simulink model "EgoCarModel"  (R2026a)
settings: Solver=FixedStepAuto
undefined symbols (not defined in the file): DiscIntNeverNeededParam, simulationParams, UT
libraries: sl_discontinuities x1
(part 1 of 2)
settings Model: Creator=rayyu  LastModifiedBy=rayyu

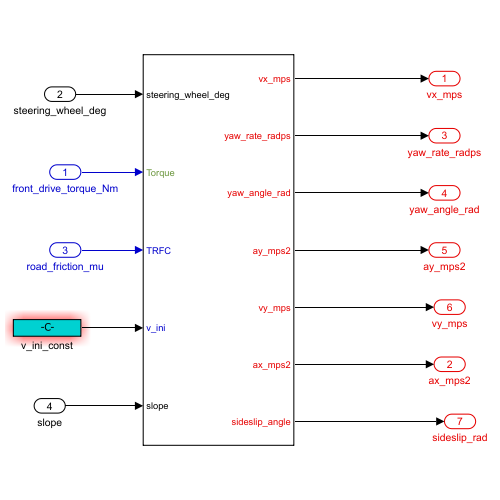
[thumbnail: Simulink's stored preview of the top-level diagram]
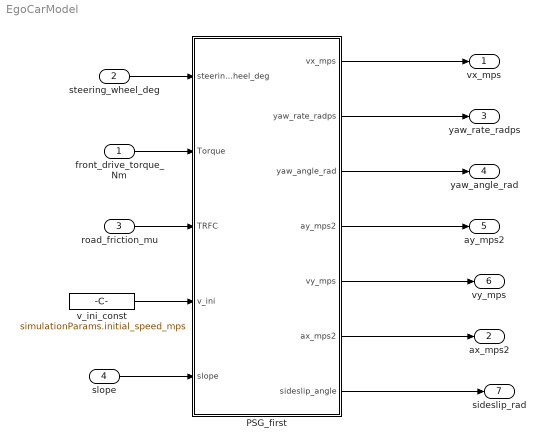
== system EgoCarModel ==
  front_drive_torque_Nm : Inport
  steering_wheel_deg : Inport  Port=2
  road_friction_mu : Inport  Port=3
  slope : Inport  Port=4
  PSG_first : Subsystem
  v_ini_const : Constant  Value=simulationParams.initial_speed_mps  VectorParams1D=off
  vx_mps : Outport
  ax_mps2 : Outport  Port=2
  yaw_rate_radps : Outport  Port=3
  yaw_angle_rad : Outport  Port=4
  ay_mps2 : Outport  Port=5
  vy_mps : Outport  Port=6
  sideslip_rad : Outport  Port=7
  wires:
  PSG_first/6(ax_mps2) -> ax_mps2/1
  road_friction_mu/1 -> PSG_first/3(TRFC)
  front_drive_torque_Nm/1 -> PSG_first/2(Torque)
  v_ini_const/1 -> PSG_first/4(v_ini)
  PSG_first/1(vx_mps) -> vx_mps/1
  steering_wheel_deg/1 -> PSG_first/1(steering_wheel_deg)
  PSG_first/2(yaw_rate_radps) -> yaw_rate_radps/1
  PSG_first/3(yaw_angle_rad) -> yaw_angle_rad/1
  PSG_first/4(ay_mps2) -> ay_mps2/1
  PSG_first/5(vy_mps) -> vy_mps/1
  PSG_first/7(sideslip_angle) -> sideslip_rad/1
  slope/1 -> PSG_first/5(slope)

== system EgoCarModel/PSG_first ==
  note: [v: 0--13--20]
      | High Frict PSG: P=75, I=125, D=15, TRFC=0.8 -->   -7.2<a<4.4
      | Low Frict  PSG: P=48, I=64,   D=12, TRFC=0.7 -->   -6.0<a<3.2
      |
      | High Frict HDV: P=27, I=27, D=9, TRFC=0.7 -->  -4.3<a<2.2
      | Low Frict  HDV: P=12, I=8,   D=6, TRFC=0.6 -->  -2.5<a<1.3
      |
      | ULMPC treat sudden drop of TRFC!
  steering_wheel_deg : Inport
  Torque : Inport  Port=2
  TRFC : Inport  Port=3
  v_ini : Inport  Port=4
  slope : Inport  Port=5
  Body Fixed Vehicle Dynamics : Subsystem
  Constant2 : Constant  Value=0
  Constant4 : Constant  Value=0
  Constant5 : Constant  Value=0
  Gain{,1..3} (4 alike) : Gain  Gain=UT.Rw
  Scope : Scope
      settings: ActiveDisplayYMinimum=-1E-6  ActiveDisplayYMaximum=1E-6
  Scope1 : Scope
      settings: ActiveDisplayYMinimum=-216705.99012  ActiveDisplayYMaximum=1.28732965782E+6  DataLoggingVariableName=ScopeData11
  Scope3 : Scope
      settings: ActiveDisplayYMinimum=-0.17988762289211868  ActiveDisplayYMaximum=0.15566007745736604  DataLoggingVariableName=ScopeData12
  Terminator : Terminator
  Vx : Scope
      settings: ActiveDisplayYMinimum=0.12308  ActiveDisplayYMaximum=39.60887  DataLoggingVariableName=ScopeData7
  ax : Scope
      settings: ActiveDisplayYMinimum=-3.96416  ActiveDisplayYMaximum=3.8969  DataLoggingVariableName=ScopeData6
  ay : Scope
      settings: ActiveDisplayYMinimum=19.63629  ActiveDisplayYMaximum=20.17019  DataLoggingVariableName=ScopeData9
  deg/rad : Gain  Gain=pi/180
  deg/rad1 : Gain  Gain=pi/180
  left/right wheel steer : Subsystem
  omegafl : Scope
      settings: ActiveDisplayYMinimum=-1.59023  ActiveDisplayYMaximum=55.33162  DataLoggingVariableName=ScopeData2
  omegafr : Scope
      settings: ActiveDisplayYMinimum=-0.02838  ActiveDisplayYMaximum=0.02291  DataLoggingVariableName=ScopeData3
  omegarl : Scope
      settings: ActiveDisplayYMinimum=-0.02838  ActiveDisplayYMaximum=0.02291  DataLoggingVariableName=ScopeData4
  omegarr : Scope
      settings: ActiveDisplayYMinimum=-0.02838  ActiveDisplayYMaximum=0.02291  DataLoggingVariableName=ScopeData5
  vy : Scope
      settings: ActiveDisplayYMinimum=19.63629  ActiveDisplayYMaximum=20.17019  DataLoggingVariableName=ScopeData10
  yaw : Scope
      settings: ActiveDisplayYMinimum=19.63629  ActiveDisplayYMaximum=20.17019
  yaw_rate : Scope
      settings: ActiveDisplayYMinimum=-0.02838  ActiveDisplayYMaximum=0.02291  DataLoggingVariableName=ScopeData8
  vx_mps : Outport
  yaw_rate_radps : Outport  Port=2
  yaw_angle_rad : Outport  Port=3
  ay_mps2 : Outport  Port=4
  vy_mps : Outport  Port=5
  ax_mps2 : Outport  Port=6
  sideslip_angle : Outport  Port=7
  wires:
  Body Fixed Vehicle Dynamics/3(omegarl) -> Gain2/1
  deg/rad1/1 -> Scope3/1, Body Fixed Vehicle Dynamics/3(deltaFR)
  Gain/1 -> omegafl/1
  Body Fixed Vehicle Dynamics/1(omegafl) -> Gain/1
  Body Fixed Vehicle Dynamics/9(ay) -> ay_mps2/1, ay/1
  v_ini/1 -> Body Fixed Vehicle Dynamics/7(V_ini)
  deg/rad/1 -> Body Fixed Vehicle Dynamics/4(deltaFL)
  slope/1 -> Body Fixed Vehicle Dynamics/5(slope)
  Body Fixed Vehicle Dynamics/12(Sideslip Angle Alpha) -> sideslip_angle/1, Scope/1
  left/right wheel steer/1(Right wheel steer ground (deg)) -> deg/rad1/1
  Body Fixed Vehicle Dynamics/10(Vy) -> vy_mps/1, vy/1
  Gain2/1 -> omegarl/1
  Body Fixed Vehicle Dynamics/8(Yaw Angle) -> yaw_angle_rad/1, yaw/1
  Body Fixed Vehicle Dynamics/11(Beta) -> Terminator/1
  Constant5/1 -> Body Fixed Vehicle Dynamics/9(vy_ini)
  steering_wheel_deg/1 -> left/right wheel steer/1(steering wheel angle deg)
  Gain3/1 -> omegarr/1
  Body Fixed Vehicle Dynamics/2(omegafr) -> Gain1/1
  Constant4/1 -> Body Fixed Vehicle Dynamics/2(Brake)
  Body Fixed Vehicle Dynamics/4(omegarr) -> Gain3/1
  Body Fixed Vehicle Dynamics/6(Vx) -> vx_mps/1, Vx/1
  Body Fixed Vehicle Dynamics/5(ax) -> ax_mps2/1, ax/1
  Constant2/1 -> Body Fixed Vehicle Dynamics/8(yaw_ini)
  left/right wheel steer/2(Left wheel steer ground (deg)) -> deg/rad/1
  Gain1/1 -> omegafr/1
  Body Fixed Vehicle Dynamics/7("Yaw Rate ") -> yaw_rate_radps/1, yaw_rate/1
  Torque/1 -> Body Fixed Vehicle Dynamics/1(Tdf), Scope1/1
  TRFC/1 -> Body Fixed Vehicle Dynamics/6(TRFC)

== system EgoCarModel/PSG_first/Body Fixed Vehicle Dynamics ==
  Tdf : Inport
  Brake : Inport  Port=2
  deltaFR : Inport  Port=3
  deltaFL : Inport  Port=4
  slope : Inport  Port=5
  TRFC : Inport  Port=6
  V_ini : Inport  Port=7
  yaw_ini : Inport  Port=8
  vy_ini : Inport  Port=9
  8dof_vehicle : Subsystem
  Brakes : Subsystem
  Bus Creator{,2..4} (4 alike) : BusCreator  Inputs=4
  Bus Creator1 : BusCreator  Inputs=8
  Bus Creator5 : BusCreator  Inputs=3
  Bus Selector : BusSelector  OutputSignals=signal1,signal2,signal3,signal4
  Constant : Constant  Value=0
  Constant1 : Constant  Value=0
  Driving Resistance Subsystem : Subsystem
  Fz : Subsystem
  Magic Formula Tire Model1 : Subsystem
  "Tire Longitudinal Center Speed " : Subsystem
  Tire Sideslip Angle : Subsystem
  To Workspace : ToWorkspace  VariableName=PSG1_FxFL  SaveFormat=Timeseries  SampleTime=-1
  To Workspace1 : ToWorkspace  VariableName=PSG1_FxRL  SaveFormat=Timeseries  SampleTime=-1
  To Workspace2 : ToWorkspace  VariableName=PSG1_FxFR  SaveFormat=Timeseries  SampleTime=-1
  To Workspace3 : ToWorkspace  VariableName=PSG1_FxRR  SaveFormat=Timeseries  SampleTime=-1
  Unit Delay : UnitDelay  SampleTime=UT.Ts_Veh
  Unit Delay1 : UnitDelay  SampleTime=UT.Ts_Veh
  deltaFL1 : InportShadow  Port=4
  deltaFL2 : InportShadow  Port=4
  deltaFR1 : InportShadow  Port=3
  deltaFR2 : InportShadow  Port=3
  lamda slip ratio : Subsystem
  omegafl : Outport  VectorParamsAs1DForOutWhenUnconnected=off
  omegafr : Outport  Port=2  VectorParamsAs1DForOutWhenUnconnected=off
  omegarl : Outport  Port=3  VectorParamsAs1DForOutWhenUnconnected=off
  omegarr : Outport  Port=4  VectorParamsAs1DForOutWhenUnconnected=off
  ax : Outport  Port=5  VectorParamsAs1DForOutWhenUnconnected=off
  Vx : Outport  Port=6  VectorParamsAs1DForOutWhenUnconnected=off
  "Yaw Rate " : Outport  Port=7  VectorParamsAs1DForOutWhenUnconnected=off
  Yaw Angle : Outport  Port=8  VectorParamsAs1DForOutWhenUnconnected=off
  ay : Outport  Port=9  VectorParamsAs1DForOutWhenUnconnected=off
  Vy : Outport  Port=10  VectorParamsAs1DForOutWhenUnconnected=off
  Beta : Outport  Port=11  VectorParamsAs1DForOutWhenUnconnected=off
  Sideslip Angle Alpha : Outport  Port=12  VectorParamsAs1DForOutWhenUnconnected=off
  wires:
  Brakes/4(Tbrr) -> 8dof_vehicle/5(Tbrr)
  Brakes/3(Tbrl) -> 8dof_vehicle/4(Tbrl)
  Brakes/2(Tbfr) -> 8dof_vehicle/3(Tbfr)
  Brakes/1(Tbfl) -> 8dof_vehicle/2(Tbfl)
  Brake/1 -> Brakes/2(brake postion)
  8dof_vehicle/14("Roll ") -> Fz/7(roll angle)
  8dof_vehicle/12(Pitch) -> Fz/4(pitch angle)
  8dof_vehicle/13(Pitch_rate) -> Fz/8(pitch rate)
  Bus Creator3/1 -> Bus Creator5/2
  deltaFR2/1 -> 8dof_vehicle/11(deltaRL)
  deltaFR1/1 -> Tire Sideslip Angle/5(deltaFR1)
  deltaFR/1 -> lamda slip ratio/10(deltaFR)
  lamda slip ratio/4(lamdarr) -> Bus Creator2/4
  lamda slip ratio/3(lamdarl) -> Bus Creator2/3
  lamda slip ratio/2(lamdafr) -> Bus Creator2/2
  lamda slip ratio/1(lamdafl) -> Bus Creator2/1
  Unit Delay/1 -> Fz/2(ax)
  Unit Delay1/1 -> Fz/5(ay)
  Magic Formula Tire Model1/4(Fy_FR) -> Bus Creator1/4
  Magic Formula Tire Model1/3(Fx_FR) -> Bus Creator1/3, To Workspace2/1
  Magic Formula Tire Model1/6(Fy_RL) -> Bus Creator1/6
  Magic Formula Tire Model1/8(Fy_RR) -> Bus Creator1/8
  Magic Formula Tire Model1/7(Fx_RR) -> Bus Creator1/7, To Workspace3/1
  Magic Formula Tire Model1/5(Fx_RL) -> Bus Creator1/5, To Workspace1/1
  deltaFL2/1 -> 8dof_vehicle/10(deltaFL)  "deltaw"
  8dof_vehicle/5(ax) -> Unit Delay/1, ax/1
  Constant/1 -> Fz/3(slope)
  Driving Resistance Subsystem/1(Fax) -> 8dof_vehicle/7(Fax), Fz/1(Fa)  "Fax"
  Constant1/1 -> Fz/6(bank angle)
  slope/1 -> 8dof_vehicle/9(slope)
  8dof_vehicle/7(Yaw Rate) -> "Tire Longitudinal Center Speed "/3(YawRate), Tire Sideslip Angle/2(Yaw Rate), "Yaw Rate "/1
  8dof_vehicle/6(Vx) -> "Tire Longitudinal Center Speed "/1(Vx), Tire Sideslip Angle/3(Vx), Driving Resistance Subsystem/1(Vx), Vx/1
  8dof_vehicle/11("Veh Sideslip, Beta") -> Tire Sideslip Angle/6(Beta), Beta/1, "Tire Longitudinal Center Speed "/4(VehSideSlip Beta)
  8dof_vehicle/9(ay) -> Unit Delay1/1, ay/1
  deltaFL1/1 -> Tire Sideslip Angle/4(deltaFL)  "deltaw"
  deltaFL/1 -> lamda slip ratio/9(deltaFL)  "deltaw"
  Driving Resistance Subsystem/2(Fr) -> 8dof_vehicle/8(Fr)
  Bus Selector/4 -> lamda slip ratio/8(Vwrr)  "<signal4>"
  Bus Selector/3 -> lamda slip ratio/7(Vwrl)  "<signal3>"
  Bus Selector/2 -> lamda slip ratio/6(Vwfr)  "<signal2>"
  Bus Selector/1 -> lamda slip ratio/5(Vwfl)  "<signal1>"
  "Tire Longitudinal Center Speed "/3(Vwrl) -> Bus Creator/3
  "Tire Longitudinal Center Speed "/1(Vwfl) -> Bus Creator/1
  "Tire Longitudinal Center Speed "/2(Vwfr) -> Bus Creator/2
  "Tire Longitudinal Center Speed "/4(Vwrr) -> Bus Creator/4
  Tire Sideslip Angle/2(alpha_fr: rad) -> Bus Creator4/2
  Tire Sideslip Angle/1(alpha_fl: rad) -> Sideslip Angle Alpha/1, Bus Creator4/1
  Tire Sideslip Angle/3(alpha_rl: rad) -> Bus Creator4/3
  Tire Sideslip Angle/4(alpha_rr: rad) -> Bus Creator4/4
  Bus Creator5/1 -> Magic Formula Tire Model1/1(VehState)
  Bus Creator4/1 -> Bus Creator5/3  "alpha"
  Bus Creator2/1 -> Brakes/1(lambda), Bus Creator5/1  "lamda"
  Fz/1(Fzfl) -> Bus Creator3/1
  Fz/2(Fzfr) -> Bus Creator3/2
  Fz/3(Fzrl) -> Bus Creator3/3
  Fz/4(Fzrr) -> Bus Creator3/4
  Magic Formula Tire Model1/1(Fx_FL) -> Bus Creator1/1, To Workspace/1
  Magic Formula Tire Model1/2(Fy_FL) -> Bus Creator1/2
  8dof_vehicle/10(Vy) -> "Tire Longitudinal Center Speed "/2(Vy), Tire Sideslip Angle/1(Vy), Vy/1
  Bus Creator1/1 -> 8dof_vehicle/6(In7)
  8dof_vehicle/8(Yaw angle) -> Yaw Angle/1
  8dof_vehicle/4(omegarr) -> lamda slip ratio/4(omegarr), omegarr/1
  8dof_vehicle/3(omegarl) -> lamda slip ratio/3(omegarl), omegarl/1
  8dof_vehicle/2(omegafr) -> omegafr/1, lamda slip ratio/2(omegafr)
  8dof_vehicle/1(omegafl) -> lamda slip ratio/1(omegafl), omegafl/1
  Tdf/1 -> 8dof_vehicle/1(Tdf)
  Bus Creator/1 -> Bus Selector/1
  TRFC/1 -> Magic Formula Tire Model1/2(TRFC)
  V_ini/1 -> 8dof_vehicle/12(V_ini)
  yaw_ini/1 -> 8dof_vehicle/13(yaw_ini)
  vy_ini/1 -> 8dof_vehicle/14(vy_ini)
  8dof_vehicle/15(Roll Rate) -> Fz/9(roll rate)

== system EgoCarModel/PSG_first/left//right wheel steer ==
  steering wheel angle deg : Inport
  Deadband Deg : DeadZone  LowerValue=-2  UpperValue=2
  Gain : Gain  Gain=0.9
  Gain1 : Gain  Gain=0.9
  Left wheel rack displacement to ground steering angle1 : Lookup_n-D  NumberOfTableDimensions=1  BreakpointsForDimension1=|  Table=|  RndMeth=Simplest
      | [-83.31
      | -80.10576923
      | -77.13888889
      | -74.38392857
      | -71.81896552
      | -69.425
      | -67.18548387
      | -65.0859375
      | -63.11363636
      | -61.25735294
      | -59.50714286
      | -57.85416667
      | -56.29054054
      | -54.80921053
      | -53.40384615
      | -52.06875
      | -50.79878049
      | -49.58928571
      | -48.43604651
      | -47.33522727
      | -46.28333333
      | -45.27717391
      | -44.31382979
      | -43.390625
      | -42.50510204
      | -41.655
      | 0
      | 41.655
      | 42.50510204
      | 43.390625
      | 44.31382979
      | 45.27717391
      | 46.28333333
      | 47.33522727
      | 48.43604651
      | 49.58928571
      | 50.79878049
      | 52.06875
      | 53.40384615
      | 54.80921053
      | 56.29054054
      | 57.85416667
      | 59.50714286
      | 61.25735294
      | 63.11363636
      | 65.0859375
      | 67.18548387
      | 69.425
      | 71.81896552
      | 74.38392857
      | 77.13888889
      | 80.10576923
      | 83.31
      | ]
      | [-39.37720355
      | -37.63494871
      | -36.07707064
      | -34.67025898
      | -33.38971041
      | -32.21639355
      | -31.13534711
      | -30.13457154
      | -29.20427963
      | -28.33637359
      | -27.52407048
      | -26.76162747
      | -26.04413644
      | -25.36736764
      | -24.72764882
      | -24.12177053
      | -23.54691095
      | -23.00057556
      | -22.48054833
      | -21.98485165
      | -21.51171342
      | -21.05953958
      | -20.62689117
      | -20.21246499
      | -19.81507719
      | -19.43364926
      | 0
      | 23.71741561
      | 24.27669186
      | 24.86323253
      | 25.47909206
      | 26.1265372
      | 26.80807528
      | 27.52648702
      | 28.28486498
      | 29.08665866
      | 29.93572777
      | 30.83640531
      | 31.7935729
      | 32.81275112
      | 33.9002085
      | 35.06309421
      | 36.30960068
      | 37.64916478
      | 39.09271935
      | 40.65301137
      | 42.34501024
      | 44.1864403
      | 46.19848973
      | 48.40677775
      | 50.84271532
      | 53.54549481
      | 56.56514507
      | ]
  Right wheel rack displacement to ground steering angle : Lookup_n-D  NumberOfTableDimensions=1  BreakpointsForDimension1=|  Table=|  RndMeth=Simplest
      | [-83.31
      | -80.10576923
      | -77.13888889
      | -74.38392857
      | -71.81896552
      | -69.425
      | -67.18548387
      | -65.0859375
      | -63.11363636
      | -61.25735294
      | -59.50714286
      | -57.85416667
      | -56.29054054
      | -54.80921053
      | -53.40384615
      | -52.06875
      | -50.79878049
      | -49.58928571
      | -48.43604651
      | -47.33522727
      | -46.28333333
      | -45.27717391
      | -44.31382979
      | -43.390625
      | -42.50510204
      | -41.655
      | 0
      | 41.655
      | 42.50510204
      | 43.390625
      | 44.31382979
      | 45.27717391
      | 46.28333333
      | 47.33522727
      | 48.43604651
      | 49.58928571
      | 50.79878049
      | 52.06875
      | 53.40384615
      | 54.80921053
      | 56.29054054
      | 57.85416667
      | 59.50714286
      | 61.25735294
      | 63.11363636
      | 65.0859375
      | 67.18548387
      | 69.425
      | 71.81896552
      | 74.38392857
      | 77.13888889
      | 80.10576923
      | 83.31
      | ]
      | [-56.56514507
      | -53.54549481
      | -50.84271532
      | -48.40677775
      | -46.19848973
      | -44.1864403
      | -42.34501024
      | -40.65301137
      | -39.09271935
      | -37.64916478
      | -36.30960068
      | -35.06309421
      | -33.9002085
      | -32.81275112
      | -31.7935729
      | -30.83640531
      | -29.93572777
      | -29.08665866
      | -28.28486498
      | -27.52648702
      | -26.80807528
      | -26.1265372
      | -25.47909206
      | -24.86323253
      | -24.27669186
      | -23.71741561
      | 0
      | 19.43364926
      | 19.81507719
      | 20.21246499
      | 20.62689117
      | 21.05953958
      | 21.51171342
      | 21.98485165
      | 22.48054833
      | 23.00057556
      | 23.54691095
      | 24.12177053
      | 24.72764882
      | 25.36736764
      | 26.04413644
      | 26.76162747
      | 27.52407048
      | 28.33637359
      | 29.20427963
      | 30.13457154
      | 31.13534711
      | 32.21639355
      | 33.38971041
      | 34.67025898
      | 36.07707064
      | 37.63494871
      | 39.37720355
      | ]
  steering wheel angle (pinion) to rack dispacement : Lookup_n-D  NumberOfTableDimensions=1  BreakpointsForDimension1=|  Table=|  RndMeth=Simplest
      BreakpointsForDimension1=|
      | [-807.1596203
      | -767.526082
      | -732.1745847
      | -700.3549602
      | -671.5005069
      | -645.1711331
      | -621.017417
      | -598.7568399
      | -578.1574816
      | -559.0264878
      | -541.2017003
      | -524.5454483
      | -508.9398532
      | -494.2832202
      | -480.4872231
      | -467.4746805
      | -455.1777777
      | -443.5366317
      | -432.4981203
      | -422.0149202
      | -412.0447096
      | -402.5495034
      | -393.495094
      | -384.8505798
      | -376.5879637
      | -368.6818104
      | 0
      | 368.6818104
      | 376.5879637
      | 384.8505798
      | 393.495094
      | 402.5495034
      | 412.0447096
      | 422.0149202
      | 432.4981203
      | 443.5366317
      | 455.1777777
      | 467.4746805
      | 480.4872231
      | 494.2832202
      | 508.9398532
      | 524.5454483
      | 541.2017003
      | 559.0264878
      | 578.1574816
      | 598.7568399
      | 621.017417
      | 645.1711331
      | 671.5005069
      | 700.3549602
      | 732.1745847
      | 767.526082
      | 807.1596203
      | ]
      Table=|
      | [-83.31
      | -80.10576923
      | -77.13888889
      | -74.38392857
      | -71.81896552
      | -69.425
      | -67.18548387
      | -65.0859375
      | -63.11363636
      | -61.25735294
      | -59.50714286
      | -57.85416667
      | -56.29054054
      | -54.80921053
      | -53.40384615
      | -52.06875
      | -50.79878049
      | -49.58928571
      | -48.43604651
      | -47.33522727
      | -46.28333333
      | -45.27717391
      | -44.31382979
      | -43.390625
      | -42.50510204
      | -41.655
      | 0
      | 41.655
      | 42.50510204
      | 43.390625
      | 44.31382979
      | 45.27717391
      | 46.28333333
      | 47.33522727
      | 48.43604651
      | 49.58928571
      | 50.79878049
      | 52.06875
      | 53.40384615
      | 54.80921053
      | 56.29054054
      | 57.85416667
      | 59.50714286
      | 61.25735294
      | 63.11363636
      | 65.0859375
      | 67.18548387
      | 69.425
      | 71.81896552
      | 74.38392857
      | 77.13888889
      | 80.10576923
      | 83.31
      | ]
  Right wheel steer ground (deg) : Outport  VectorParamsAs1DForOutWhenUnconnected=off
  Left wheel steer ground (deg) : Outport  Port=2  VectorParamsAs1DForOutWhenUnconnected=off
  wires:
  Deadband Deg/1 -> steering wheel angle (pinion) to rack dispacement/1
  Gain1/1 -> Left wheel steer ground (deg)/1
  Gain/1 -> Right wheel steer ground (deg)/1
  Left wheel rack displacement to ground steering angle1/1 -> Gain1/1
  Right wheel rack displacement to ground steering angle/1 -> Gain/1
  steering wheel angle (pinion) to rack dispacement/1 -> Right wheel rack displacement to ground steering angle/1, Left wheel rack displacement to ground steering angle1/1
  steering wheel angle deg/1 -> Deadband Deg/1

== system EgoCarModel/PSG_first/Body Fixed Vehicle Dynamics/8dof_vehicle ==
  Tdf : Inport
  Tbfl : Inport  Port=2
  Tbfr : Inport  Port=3
  Tbrl : Inport  Port=4
  Tbrr : Inport  Port=5
  In7 : Inport  Port=6
  Fax : Inport  Port=7
  Fr : Inport  Port=8
  slope : Inport  Port=9
  deltaFL : Inport  Port=10
  deltaRL : Inport  Port=11
  V_ini : Inport  Port=12
  yaw_ini : Inport  Port=13
  vy_ini : Inport  Port=14
  4tyre_torque : Subsystem
  Bus Selector1 : BusSelector  OutputSignals=Fx_FL,Fx_FR,Fx_RL,Fx_RR,Fy_FL,Fy_FR
  Bus Selector2 : BusSelector  OutputSignals=Fy_FL,Fy_FR,Fy_RL,Fy_RR,Fx_FL,Fx_FR
  Bus Selector3 : BusSelector  OutputSignals=Fx_FL,Fx_FR,Fx_RL,Fx_RR
  Bus Selector4 : BusSelector  OutputSignals=Fy_FL,Fy_FR,Fy_RL,Fy_RR,Fx_FL,Fx_FR,Fx_RL,Fx_RR
  Constant1 : Constant  Value=0
  Gain2 : Gain  Gain=-1
  "Pitch " : Subsystem
  Roll : Subsystem
  Switch{,1..3} (4 alike) : Switch  SaturateOnIntegerOverflow=off  InputSameDT=off
  Yaw Dynamics : Subsystem
  deltaFL1 : InportShadow  Port=10
  deltaFL2 : InportShadow  Port=10
  deltaRL1 : InportShadow  Port=11
  deltaRL2 : InportShadow  Port=11
  lateral : Subsystem
  longitudinal : Subsystem
  omegafl : Outport  VectorParamsAs1DForOutWhenUnconnected=off
  omegafr : Outport  Port=2  VectorParamsAs1DForOutWhenUnconnected=off
  omegarl : Outport  Port=3  VectorParamsAs1DForOutWhenUnconnected=off
  omegarr : Outport  Port=4  VectorParamsAs1DForOutWhenUnconnected=off
  ax : Outport  Port=5  VectorParamsAs1DForOutWhenUnconnected=off
  Vx : Outport  Port=6  VectorParamsAs1DForOutWhenUnconnected=off
  Yaw Rate : Outport  Port=7  VectorParamsAs1DForOutWhenUnconnected=off
  Yaw angle : Outport  Port=8  VectorParamsAs1DForOutWhenUnconnected=off
  ay : Outport  Port=9  VectorParamsAs1DForOutWhenUnconnected=off
  Vy : Outport  Port=10  VectorParamsAs1DForOutWhenUnconnected=off
  "Veh Sideslip, Beta" : Outport  Port=11  VectorParamsAs1DForOutWhenUnconnected=off
  Pitch : Outport  Port=12  VectorParamsAs1DForOutWhenUnconnected=off
  Pitch_rate : Outport  Port=13  VectorParamsAs1DForOutWhenUnconnected=off
  "Roll " : Outport  Port=14  VectorParamsAs1DForOutWhenUnconnected=off
  Roll Rate : Outport  Port=15  VectorParamsAs1DForOutWhenUnconnected=off
  wires:
  Switch/1 -> 4tyre_torque/4(Tbrl)
  Switch1/1 -> 4tyre_torque/2(Tbfl)
  Bus Selector3/4 -> 4tyre_torque/9(Fxrr)  "<Fx_RR>"
  Bus Selector3/3 -> 4tyre_torque/8(Fxrl)  "<Fx_RL>"
  Bus Selector3/2 -> 4tyre_torque/7(Fxfr)  "<Fx_FR>"
  Bus Selector3/1 -> 4tyre_torque/6(Fxfl)  "<Fx_FL>"
  Switch2/1 -> 4tyre_torque/3(Tbfr)
  Switch3/1 -> 4tyre_torque/5(Tbrr)
  Tbrr/1 -> Switch3/3
  Tbfr/1 -> Switch2/3
  Constant1/1 -> Switch3/1, Switch/1, Switch2/1, Switch1/1
  Tbfl/1 -> Switch1/3
  Gain2/1 -> Switch3/2, Switch2/2, Switch1/2, Switch/2
  Tdf/1 -> 4tyre_torque/1(Tdf)
  4tyre_torque/4(omega_rr) -> omegarr/1
  4tyre_torque/3(omega_rl) -> omegarl/1
  4tyre_torque/2(omega_fr) -> omegafr/1
  Tbrl/1 -> Switch/3
  4tyre_torque/1(omega_fl) -> omegafl/1
  "Pitch "/3(pitch Accel) -> longitudinal/15(pitch_accel)
  Yaw Dynamics/3(Yaw Accel) -> lateral/16(yaw_accel), longitudinal/20(yaw_accel)
  Roll/3(Roll Accel) -> lateral/14(roll_accel), longitudinal/18(roll_accel)
  "Pitch "/1(pitch_rate) -> Pitch_rate/1, Roll/4(pitch_rate), lateral/11(pitch_rate), longitudinal/14(pitch_rate)
  "Pitch "/2(pitch) -> Roll/2(pitch), Yaw Dynamics/16("pitch "), lateral/10(pitch), longitudinal/13(pitch), Pitch/1
  Roll/1(roll_rate) -> "Pitch "/4(roll_rate), lateral/13(roll_rate), longitudinal/17(roll_rate), Roll Rate/1
  Roll/2(roll) -> "Roll "/1, Yaw Dynamics/15(roll), "Pitch "/2(roll), lateral/12(roll), longitudinal/16(roll)
  lateral/4(Fy) -> Yaw Dynamics/14(Fy), Roll/1(Fy)
  longitudinal/3(Fx) -> "Pitch "/1(Fx), Yaw Dynamics/13(Fx)
  deltaRL1/1 -> Yaw Dynamics/12(In11)
  deltaFL1/1 -> Yaw Dynamics/11(In10)
  Bus Selector4/8 -> Yaw Dynamics/10(In8)  "<Fx_RR>"
  Bus Selector4/7 -> Yaw Dynamics/9(In7)  "<Fx_RL>"
  Bus Selector4/6 -> Yaw Dynamics/8(In2)  "<Fx_FR>"
  Bus Selector4/5 -> Yaw Dynamics/7(In1)  "<Fx_FL>"
  Bus Selector4/4 -> Yaw Dynamics/6(In6)  "<Fy_RR>"
  Bus Selector4/3 -> Yaw Dynamics/5(In5)  "<Fy_RL>"
  Bus Selector4/2 -> Yaw Dynamics/4(In4)  "<Fy_FR>"
  Bus Selector4/1 -> Yaw Dynamics/3(In3)  "<Fy_FL>"
  Yaw Dynamics/1(Yaw angle) -> Yaw angle/1
  Yaw Dynamics/2(Yaw Rate) -> "Pitch "/3(yaw_rate), lateral/15(yaw_rate), longitudinal/19(yaw_rate), Roll/3(yaw_rate), Yaw Rate/1
  deltaRL2/1 -> lateral/9(deltaFR)
  deltaRL/1 -> longitudinal/12(deltaFR)
  longitudinal/1(ax) -> ax/1
  Bus Selector2/1 -> lateral/1(In7)  "<Fy_FL>"
  Bus Selector2/6 -> lateral/6(In12)  "<Fx_FR>"
  Bus Selector2/2 -> lateral/2(In8)  "<Fy_FR>"
  Bus Selector2/3 -> lateral/3(In9)  "<Fy_RL>"
  Bus Selector2/5 -> lateral/5(In11)  "<Fx_FL>"
  Bus Selector2/4 -> lateral/4(In10)  "<Fy_RR>"
  deltaFL2/1 -> lateral/8(deltaFL)
  lateral/3(Veh Sideslip angle,Beta1) -> Yaw Dynamics/2(Beta), "Veh Sideslip, Beta"/1
  longitudinal/2(Vx) -> lateral/7(Vx1), Yaw Dynamics/1(Vx), Gain2/1, Vx/1
  Bus Selector1/6 -> longitudinal/6(In4)  "<Fy_FR>"
  Bus Selector1/5 -> longitudinal/5(In3)  "<Fy_FL>"
  deltaFL/1 -> longitudinal/11(deltaFL)
  lateral/1(ay1) -> ay/1
  slope/1 -> longitudinal/9(slope)
  Fr/1 -> longitudinal/8(Fr)
  Bus Selector1/4 -> longitudinal/4(In6)  "<Fx_RR>"
  Bus Selector1/3 -> longitudinal/3(In5)  "<Fx_RL>"
  Bus Selector1/1 -> longitudinal/1(In1)  "<Fx_FL>"
  Bus Selector1/2 -> longitudinal/2(In2)  "<Fx_FR>"
  In7/1 -> Bus Selector2/1, Bus Selector1/1, Bus Selector3/1, Bus Selector4/1
  lateral/2(Vy1) -> longitudinal/10(Vy), Vy/1
  Fax/1 -> longitudinal/7(Fax)
  yaw_ini/1 -> Yaw Dynamics/17(yaw_ini)
  vy_ini/1 -> lateral/17(vy_ini)
  V_ini/1 -> 4tyre_torque/10(V_ini), longitudinal/21(V_ini)

== system EgoCarModel/PSG_first/Body Fixed Vehicle Dynamics/Brakes ==
  note: 0-100
  lambda : Inport
  brake postion : Inport  Port=2
  "-1 " : Gain  Commented=on  Gain=-1
  Bus Selector : BusSelector  OutputSignals=signal1,signal2,signal3,signal4
  Constant : Constant  Commented=on  Value=0
  Constant1 : Constant  Value=0
  Constant2 : Constant  Value=0
  Delay{,1..3} (4 alike) : Delay  DelayLength=6  InitialCondition=0
  From : From  Commented=on  GotoTag=Des_Torque
  Front Brake Torque vs Pressure : Gain  Gain=300
  Front Prop Valve : Gain
  Rear Brake Torque vs Pressure1 : Gain  Gain=150
  Rear Prop Valve : Lookup_n-D  NumberOfTableDimensions=1  BreakpointsForDimension1=[0 2.5 3.5]  Table=[0 2.5 2.8]  DiagnosticForOutOfRangeInput=Warning  RndMeth=Simplest
  Switch : Switch  Commented=on  SaturateOnIntegerOverflow=off  InputSameDT=off
  Switch1 : Switch  Threshold=0.12  SaturateOnIntegerOverflow=off  InputSameDT=off
  Switch2 : Switch  Threshold=0.12  SaturateOnIntegerOverflow=off  InputSameDT=off
  Switch3 : Switch  Threshold=0.15  SaturateOnIntegerOverflow=off  InputSameDT=off
  Switch4 : Switch  Threshold=0.15  SaturateOnIntegerOverflow=off  InputSameDT=off
  Terminator : Terminator  Commented=on
  brake position to master cylinder pressure : Gain  Gain=.0345
  Tbfl : Outport  VectorParamsAs1DForOutWhenUnconnected=off
  Tbfr : Outport  Port=2  VectorParamsAs1DForOutWhenUnconnected=off
  Tbrl : Outport  Port=3  VectorParamsAs1DForOutWhenUnconnected=off
  Tbrr : Outport  Port=4  VectorParamsAs1DForOutWhenUnconnected=off
  wires:
  Rear Prop Valve/1 -> Rear Brake Torque vs Pressure1/1
  Rear Brake Torque vs Pressure1/1 -> Switch4/3, Switch3/3
  Switch1/1 -> Delay/1
  Switch2/1 -> Delay1/1
  Switch3/1 -> Delay2/1
  Switch4/1 -> Delay3/1
  Bus Selector/1 -> Switch1/2  "<signal1>"
  Constant1/1 -> Switch2/1, Switch1/1
  Front Brake Torque vs Pressure/1 -> Switch2/3, Switch1/3
  Bus Selector/2 -> Switch2/2  "<signal2>"
  Bus Selector/3 -> Switch3/2  "<signal3>"
  Bus Selector/4 -> Switch4/2  "<signal4>"
  Constant2/1 -> Switch4/1, Switch3/1
  Front Prop Valve/1 -> Front Brake Torque vs Pressure/1
  brake position to master cylinder pressure/1 -> Rear Prop Valve/1, Front Prop Valve/1
  Constant/1 -> Switch/1
  From/1 -> "-1 "/1, Switch/2
  "-1 "/1 -> Switch/3
  brake postion/1 -> brake position to master cylinder pressure/1
  Switch/1 -> Terminator/1
  lambda/1 -> Bus Selector/1
  Delay/1 -> Tbfl/1
  Delay1/1 -> Tbfr/1
  Delay2/1 -> Tbrl/1
  Delay3/1 -> Tbrr/1

== system EgoCarModel/PSG_first/Body Fixed Vehicle Dynamics/Driving Resistance Subsystem ==
  Vx : Inport
  Aerodynamic Resistance : Subsystem
  Rolling resistance : Subsystem
  Fax : Outport  VectorParamsAs1DForOutWhenUnconnected=off
  Fr : Outport  Port=2  VectorParamsAs1DForOutWhenUnconnected=off
  wires:
  Rolling resistance/1(Fr) -> Fr/1
  Aerodynamic Resistance/1(Fa) -> Fax/1
  Vx/1 -> Rolling resistance/1(Vx), Aerodynamic Resistance/1(Vx)

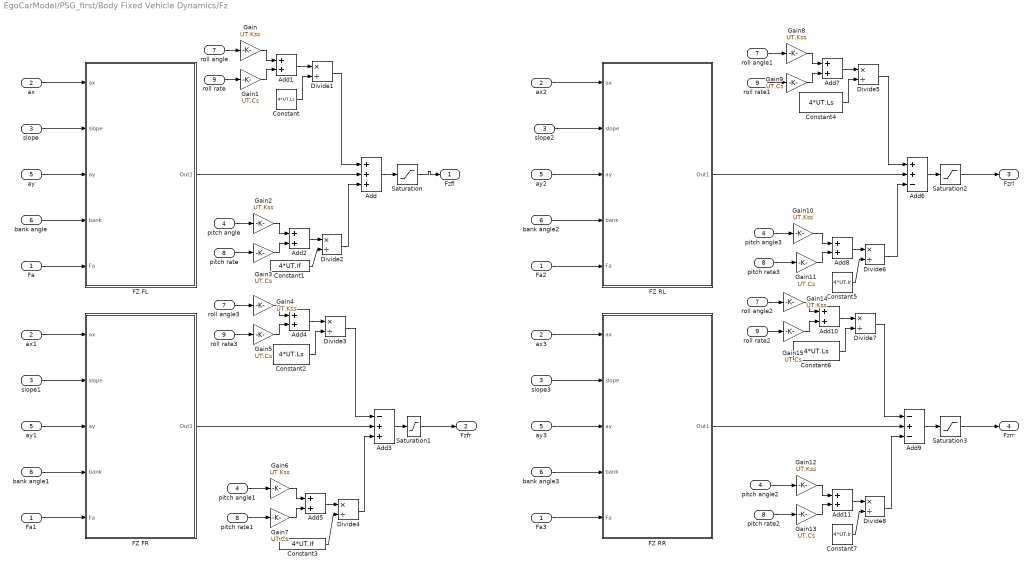
== system EgoCarModel/PSG_first/Body Fixed Vehicle Dynamics/Fz ==
  Fa : Inport
  ax : Inport  Port=2
  slope : Inport  Port=3
  pitch angle : Inport  Port=4
  ay : Inport  Port=5
  bank angle : Inport  Port=6
  roll angle : Inport  Port=7
  pitch rate : Inport  Port=8
  roll rate : Inport  Port=9
  Add : Sum  Inputs=+++
  Add{1..2,4..5,7..8,10..11} (8 alike) : Sum
  Add3 : Sum  Inputs=-++
  Add6 : Sum  Inputs=++-
  Add9 : Sum  Inputs=-+-
  Constant{,2,4,6} (4 alike) : Constant  Value=4*UT.Ls
  Constant1 : Constant  Value=4*UT.lf
  Constant3 : Constant  Value=4*UT.lf
  Constant5 : Constant  Value=4*UT.lr
  Constant7 : Constant  Value=4*UT.lr
  Divide{1..8} (8 alike) : Product  Inputs=*/
  FZ FL : Subsystem
  FZ FR : Subsystem
  FZ RL : Subsystem
  FZ RR : Subsystem
  Fa1 : InportShadow
  Fa2 : InportShadow
  Fa3 : InportShadow
  Gain{,2,4,6,8,10,12,14} (8 alike) : Gain  Gain=UT.Kss
  Gain{1,3,5,7,9,11,13,15} (8 alike) : Gain  Gain=UT.Cs
  Saturation{,1..3} (4 alike) : Saturate  UpperLimit=10000  LowerLimit=100
  ax1 : InportShadow  Port=2
  ax2 : InportShadow  Port=2
  ax3 : InportShadow  Port=2
  ay1 : InportShadow  Port=5
  ay2 : InportShadow  Port=5
  ay3 : InportShadow  Port=5
  bank angle1 : InportShadow  Port=6
  bank angle2 : InportShadow  Port=6
  bank angle3 : InportShadow  Port=6
  pitch angle1 : InportShadow  Port=4
  pitch angle2 : InportShadow  Port=4
  pitch angle3 : InportShadow  Port=4
  pitch rate1 : InportShadow  Port=8
  pitch rate2 : InportShadow  Port=8
  pitch rate3 : InportShadow  Port=8
  roll angle1 : InportShadow  Port=7
  roll angle2 : InportShadow  Port=7
  roll angle3 : InportShadow  Port=7
  roll rate1 : InportShadow  Port=9
  roll rate2 : InportShadow  Port=9
  roll rate3 : InportShadow  Port=9
  slope1 : InportShadow  Port=3
  slope2 : InportShadow  Port=3
  slope3 : InportShadow  Port=3
  Fzfl : Outport  VectorParamsAs1DForOutWhenUnconnected=off
  Fzfr : Outport  Port=2  VectorParamsAs1DForOutWhenUnconnected=off
  Fzrl : Outport  Port=3  VectorParamsAs1DForOutWhenUnconnected=off
  Fzrr : Outport  Port=4  VectorParamsAs1DForOutWhenUnconnected=off
  wires:
  Divide6/1 -> Add6/3
  Divide8/1 -> Add9/3
  Divide2/1 -> Add/3
  Divide4/1 -> Add3/3
  Saturation3/1 -> Fzrr/1
  Saturation2/1 -> Fzrl/1
  Saturation1/1 -> Fzfr/1
  Saturation/1 -> Fzfl/1
  Divide7/1 -> Add9/1
  Divide5/1 -> Add6/1
  Divide3/1 -> Add3/1
  Divide1/1 -> Add/1
  Add9/1 -> Saturation3/1
  Add6/1 -> Saturation2/1
  Add3/1 -> Saturation1/1
  pitch rate2/1 -> Gain13/1
  pitch angle2/1 -> Gain12/1
  Constant7/1 -> Divide8/2
  Add11/1 -> Divide8/1
  Gain12/1 -> Add11/1
  Gain13/1 -> Add11/2
  FZ RR/1(Out1) -> Add9/2
  Constant6/1 -> Divide7/2
  Add10/1 -> Divide7/1
  Gain14/1 -> Add10/1
  Gain15/1 -> Add10/2
  roll rate2/1 -> Gain15/1
  roll angle2/1 -> Gain14/1
  pitch rate3/1 -> Gain11/1
  pitch angle3/1 -> Gain10/1
  Constant5/1 -> Divide6/2
  Add8/1 -> Divide6/1
  Gain10/1 -> Add8/1
  Gain11/1 -> Add8/2
  FZ RL/1(Out1) -> Add6/2
  Constant4/1 -> Divide5/2
  Add7/1 -> Divide5/1
  Gain8/1 -> Add7/1
  Gain9/1 -> Add7/2
  roll rate1/1 -> Gain9/1
  roll angle1/1 -> Gain8/1
  pitch rate1/1 -> Gain7/1
  pitch angle1/1 -> Gain6/1
  Constant3/1 -> Divide4/2
  Add5/1 -> Divide4/1
  Gain6/1 -> Add5/1
  Gain7/1 -> Add5/2
  FZ FR/1(Out1) -> Add3/2
  Constant2/1 -> Divide3/2
  Add4/1 -> Divide3/1
  Gain4/1 -> Add4/1
  Gain5/1 -> Add4/2
  roll rate3/1 -> Gain5/1
  roll angle3/1 -> Gain4/1
  pitch rate/1 -> Gain3/1
  pitch angle/1 -> Gain2/1
  Constant1/1 -> Divide2/2
  Add2/1 -> Divide2/1
  Gain2/1 -> Add2/1
  Gain3/1 -> Add2/2
  Add/1 -> Saturation/1
  FZ FL/1(Out1) -> Add/2
  Constant/1 -> Divide1/2
  Add1/1 -> Divide1/1
  Gain/1 -> Add1/1
  Gain1/1 -> Add1/2
  roll rate/1 -> Gain1/1
  roll angle/1 -> Gain/1
  Fa1/1 -> FZ FR/5(Fa)
  bank angle1/1 -> FZ FR/4(bank)
  ay1/1 -> FZ FR/3(ay)
  ax1/1 -> FZ FR/1(ax)
  slope1/1 -> FZ FR/2(slope)
  bank angle3/1 -> FZ RR/4(bank)
  ax3/1 -> FZ RR/1(ax)
  Fa3/1 -> FZ RR/5(Fa)
  ay3/1 -> FZ RR/3(ay)
  slope3/1 -> FZ RR/2(slope)
  Fa2/1 -> FZ RL/5(Fa)
  ax2/1 -> FZ RL/1(ax)
  bank angle2/1 -> FZ RL/4(bank)
  slope2/1 -> FZ RL/2(slope)
  ay2/1 -> FZ RL/3(ay)
  bank angle/1 -> FZ FL/4(bank)
  Fa/1 -> FZ FL/5(Fa)
  ay/1 -> FZ FL/3(ay)
  ax/1 -> FZ FL/1(ax)
  slope/1 -> FZ FL/2(slope)

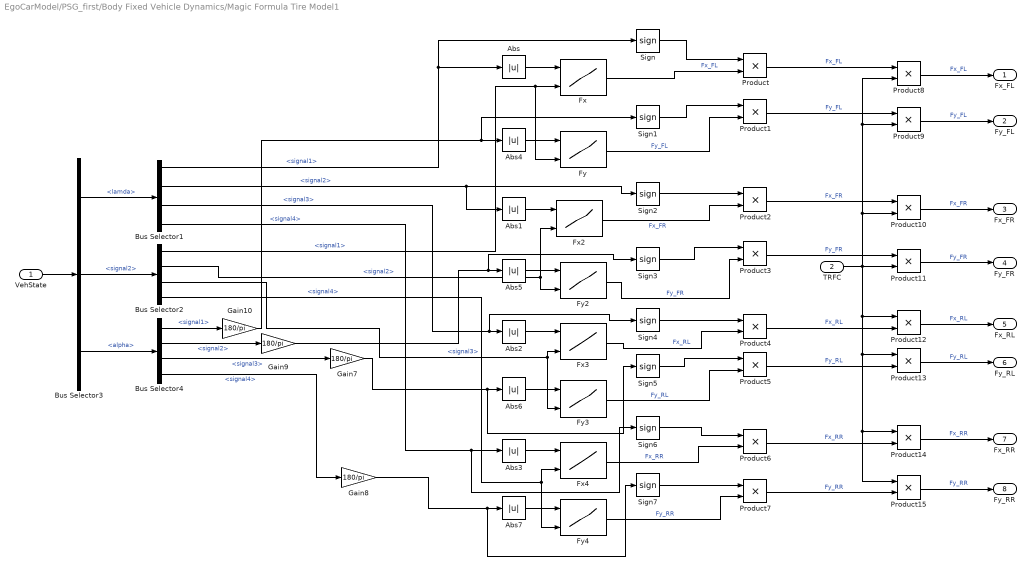
== system EgoCarModel/PSG_first/Body Fixed Vehicle Dynamics/Magic Formula Tire Model1 ==
  VehState : Inport
  TRFC : Inport  Port=2
  Abs{,1..7} (8 alike) : Abs  SaturateOnIntegerOverflow=off
  Bus Selector1 : BusSelector  OutputSignals=signal1,signal2,signal3,signal4
  Bus Selector2 : BusSelector  OutputSignals=signal1,signal2,signal3,signal4
  Bus Selector3 : BusSelector  OutputSignals=lamda,signal2,alpha
  Bus Selector4 : BusSelector  OutputSignals=signal1,signal2,signal3,signal4
  Fx{,2..4} (4 alike) : Lookup_n-D  BreakpointsForDimension1=[0,0.02,0.04,0.06,0.08,0.1,0.12,0.14,0.16,0.18,0.2,0.25,0.3,0.4,0.5,0.6,0.7,0.8,0.9,1]  BreakpointsForDimension2=[0,2105,3995,6120,7900,10100]  Table=reshape([0,0,0,0,0,0,0,0,0,0,0,0,0,0,0,0,0,0,0,0,0,926.741,1701.43,2240.07,2548.95,2689.78,2729.82,2717.36,2680.7,2634.75,2586.89,2476.95,2388.22,2262.94,2181.64,2125.47,2084.58,2053.55,2029.26,2029.26,0,1853.48,3402.86,4480.13,5097.92,5379.54,5459.63,5434.73,5361.4,5269.5,5173.78,4953.9,4776.46,4525.87,4363.28,4250.95,4169.16,4107.12,4058.51,4058.51,0,2780.22,5104.29,6720.21,7646.88,8069.32,8189.45,8152.09,8042.1,7904.24,7760.68,7430.85,7164.69,6788.82,6544.93,6376.42,6253.75,6160.67,6087.76,6087.76,0,3706.97,6805.72,8960.27,10195.8,10759.1,10919.3,10869.4,10722.8,10539,10347.6,9907.79,9552.92,9051.76,8726.56,8501.91,8338.33,8214.24,8117.01,8117.01,0,4633.7,8507.15,11200.3,12744.8,13448.8,13649.1,13586.8,13403.5,13173.7,12934.4,12384.7,11941.1,11314.7,10908.2,10627.4,10422.9,10267.8,10146.3,10146.3],20,6)  RndMeth=Simplest
      settings: InputPortMap=u0,u1
  Fy{,2..4} (4 alike) : Lookup_n-D  BreakpointsForDimension1=[0,0.5,1,1.5,2,2.5,3,3.5,4,4.5,5,5.5,6,6.5,7,7.5,8,8.5,9,9.5,10,12,14,16,18,20]  BreakpointsForDimension2=[0,1725,3500,6100,6950,9005]  Table=reshape([0,0,0,0,0,0,0,0,0,0,0,0,0,0,0,0,0,0,0,0,0,0,0,0,0,0,0,444.357,843.546,1162.09,1403.45,1580.72,1707.08,1795.66,1859.6,1893.83,1904.16,1896.19,1875.03,1845.3,1810.95,1775.12,1740.18,1707.8,1678.67,1653.27,1631.62,1574.53,1546.58,1531.91,1523.64,1523.64,0,894.186,1694.5,2327.41,2800.6,3142.1,3379.93,3542.12,3656.67,3713.24,3724.46,3701.92,3656.45,3597,3531.15,3464.91,3402.12,3345.23,3295.32,3252.61,3216.48,3123.37,3078,3054.18,3040.4,3040.4,0,1293.54,2452.99,3373.13,4064.18,4565.24,4915.41,5153.78,5319.43,5402.64,5422.23,5395.45,5337.38,5261.2,5177.14,5092.89,5013.56,4942.1,4879.5,4825.96,4780.78,4662.96,4604.6,4573.3,4554.99,4554.99,0,1601.93,3047.78,4214.48,5111.02,5779.43,6261.69,6599.82,6835.85,6968.31,7019.99,7011.91,6962.7,6887.9,6800.2,6709.15,6621.16,6540.06,6467.91,6405.21,6351.47,6207.67,6133.95,6093.89,6070.17,6070.17,0,1784.39,3417.9,4780.29,5873.77,6731.16,7385.32,7869.06,8215.23,8439.3,8564.79,8613.61,8605.54,8557.9,8485.17,8398.94,8308.19,8219.02,8135.36,8059.17,7991.56,7798.93,7693.72,7634.76,7599.62,7599.62],26,6)  RndMeth=Simplest
      settings: InputPortMap=u0,u1
  Gain{7..10} (4 alike) : Gain  Gain=180/pi  SaturateOnIntegerOverflow=on  SampleTime=UT.Ts_Veh  OutDataTypeStr=Inherit: Same as input  ParamDataTypeStr=Inherit: Same as input
  Product{,1..15} (16 alike) : Product
  Sign{,1..7} (8 alike) : Signum
  Fx_FL : Outport  VectorParamsAs1DForOutWhenUnconnected=off
  Fy_FL : Outport  Port=2  VectorParamsAs1DForOutWhenUnconnected=off
  Fx_FR : Outport  Port=3  VectorParamsAs1DForOutWhenUnconnected=off
  Fy_FR : Outport  Port=4  VectorParamsAs1DForOutWhenUnconnected=off
  Fx_RL : Outport  Port=5  VectorParamsAs1DForOutWhenUnconnected=off
  Fy_RL : Outport  Port=6  VectorParamsAs1DForOutWhenUnconnected=off
  Fx_RR : Outport  Port=7  VectorParamsAs1DForOutWhenUnconnected=off
  Fy_RR : Outport  Port=8  VectorParamsAs1DForOutWhenUnconnected=off
  wires:
  Product15/1 -> Fy_RR/1  "Fy_RR"
  Product14/1 -> Fx_RR/1  "Fx_RR"
  Product13/1 -> Fy_RL/1  "Fy_RL"
  Product12/1 -> Fx_RL/1  "Fx_RL"
  Product11/1 -> Fy_FR/1  "Fy_FR"
  Product10/1 -> Fx_FR/1  "Fx_FR"
  Product9/1 -> Fy_FL/1  "Fy_FL"
  Product8/1 -> Fx_FL/1  "Fx_FL"
  Fy4/1 -> Product7/2  "Fy_RR"
  Sign7/1 -> Product7/1
  Product6/1 -> Product14/2  "Fx_RR"
  Fx4/1 -> Product6/2  "Fx_RR"
  Sign6/1 -> Product6/1
  Fy3/1 -> Product5/2  "Fy_RL"
  Sign5/1 -> Product5/1
  Product4/1 -> Product12/2  "Fx_RL"
  Fx3/1 -> Product4/2  "Fx_RL"
  Sign4/1 -> Product4/1
  Fy2/1 -> Product3/2  "Fy_FR"
  Sign3/1 -> Product3/1
  Product2/1 -> Product10/1  "Fx_FR"
  Fx2/1 -> Product2/2  "Fx_FR"
  Sign2/1 -> Product2/1
  Fy/1 -> Product1/2  "Fy_FL"
  Sign1/1 -> Product1/1
  Product/1 -> Product8/1  "Fx_FL"
  Fx/1 -> Product/2  "Fx_FL"
  Sign/1 -> Product/1
  Gain8/1 -> Abs7/1, Sign7/1
  Gain7/1 -> Abs6/1, Sign5/1
  Gain9/1 -> Abs5/1, Sign3/1
  Gain10/1 -> Abs4/1, Sign1/1
  Abs7/1 -> Fy4/1
  Abs6/1 -> Fy3/1
  Abs5/1 -> Fy2/1
  Abs4/1 -> Fy/1
  Bus Selector2/4 -> Fx4/2, Fy4/2  "<signal4>"
  Abs3/1 -> Fx4/1
  Bus Selector2/3 -> Fx3/2, Fy3/2  "<signal3>"
  Bus Selector2/2 -> Fx2/2, Fy2/2  "<signal2>"
  Abs2/1 -> Fx3/1
  Abs1/1 -> Fx2/1
  Bus Selector2/1 -> Fx/2, Fy/2  "<signal1>"
  Abs/1 -> Fx/1
  Bus Selector1/3 -> Abs2/1, Sign4/1  "<signal3>"
  Bus Selector1/2 -> Abs1/1, Sign2/1  "<signal2>"
  Bus Selector1/1 -> Abs/1, Sign/1  "<signal1>"
  VehState/1 -> Bus Selector3/1
  Bus Selector1/4 -> Abs3/1, Sign6/1  "<signal4>"
  Bus Selector4/1 -> Gain10/1  "<signal1>"
  Bus Selector4/2 -> Gain9/1  "<signal2>"
  Bus Selector4/3 -> Gain7/1  "<signal3>"
  Bus Selector4/4 -> Gain8/1  "<signal4>"
  Bus Selector3/1 -> Bus Selector1/1  "<lamda>"
  Bus Selector3/2 -> Bus Selector2/1  "<signal2>"
  Bus Selector3/3 -> Bus Selector4/1  "<alpha>"
  Product3/1 -> Product11/1  "Fy_FR"
  Product5/1 -> Product13/2  "Fy_RL"
  Product7/1 -> Product15/2  "Fy_RR"
  Product1/1 -> Product9/1  "Fy_FL"
  TRFC/1 -> Product15/1, Product14/1, Product13/1, Product12/1, Product8/2, Product9/2, Product10/2, Product11/2

== system EgoCarModel/PSG_first/Body Fixed Vehicle Dynamics/Tire Longitudinal Center Speed  ==
  note: Vcg
  Vx : Inport
  Vy : Inport  Port=2
  YawRate : Inport  Port=3
  VehSideSlip Beta : Inport  Port=4
  Add{,1,4,6,8} (5 alike) : Sum  SampleTime=UT.Ts_Veh
  Add2 : Sum  Inputs=+-  SampleTime=UT.Ts_Veh
  Add3 : Sum  Inputs=-+  SampleTime=UT.Ts_Veh
  Add5 : Sum  Inputs=-+  SampleTime=UT.Ts_Veh
  Add7 : Sum  Inputs=+-  SampleTime=UT.Ts_Veh
  Gain : Gain
  "Ls " : Constant  Value=UT.Ls
  Math Function : Math  Operator=square  SignedPower=on  SampleTime=UT.Ts_Veh
  Math Function1 : Math  Operator=square  SignedPower=on  SampleTime=UT.Ts_Veh
  Product{,1..5} (6 alike) : Product  SampleTime=UT.Ts_Veh
  Sqrt : Sqrt  SampleTime=UT.Ts_Veh
  lf : Constant  Value=UT.lf
  lr : Constant  Value=UT.lr
  Vwfl : Outport  VectorParamsAs1DForOutWhenUnconnected=off
  Vwfr : Outport  Port=2  VectorParamsAs1DForOutWhenUnconnected=off
  Vwrl : Outport  Port=3  VectorParamsAs1DForOutWhenUnconnected=off
  Vwrr : Outport  Port=4  VectorParamsAs1DForOutWhenUnconnected=off
  wires:
  Gain/1 -> Product3/1, Product/1
  Add8/1 -> Vwrr/1
  Product5/1 -> Add8/2
  Add5/1 -> Product5/2
  Add7/1 -> Vwrl/1
  Product4/1 -> Add7/2
  Add6/1 -> Product4/2
  Product3/1 -> Add6/2, Add5/1
  lr/1 -> Product3/2
  Add1/1 -> Vwfr/1
  Product2/1 -> Add1/2
  Add4/1 -> Product2/2
  Add2/1 -> Vwfl/1
  Product1/1 -> Add2/2
  Sqrt/1 -> Add2/1, Add1/1, Add7/1, Add8/1
  Add3/1 -> Product1/2
  "Ls "/1 -> Add3/2, Add4/2, Add6/1, Add5/2
  Product/1 -> Add3/1, Add4/1
  VehSideSlip Beta/1 -> Gain/1
  lf/1 -> Product/2
  YawRate/1 -> Product1/1, Product2/1, Product4/1, Product5/1
  Add/1 -> Sqrt/1
  Math Function1/1 -> Add/2
  Math Function/1 -> Add/1
  Vx/1 -> Math Function/1
  Vy/1 -> Math Function1/1

== system EgoCarModel/PSG_first/Body Fixed Vehicle Dynamics/Tire Sideslip Angle ==
  Vy : Inport
  Yaw Rate : Inport  Port=2
  Vx : Inport  Port=3
  deltaFL : Inport  Port=4
  deltaFR1 : Inport  Port=5
  Beta : Inport  Port=6
  Add : Sum  SampleTime=UT.Ts_Veh
  Add1 : Sum  Inputs=--+  SampleTime=UT.Ts_Veh
  Add2 : Sum  Inputs=-+  SampleTime=UT.Ts_Veh
  Add4 : Sum  Inputs=--+  SampleTime=UT.Ts_Veh
  Constant : Constant  Value=UT.lf
  Constant1 : Constant  Value=UT.lr
  Constant2 : Constant  Value=0.001
  Constant{3..6} (4 alike) : Constant  Value=0
  Divide : Product  Inputs=*/  SampleTime=UT.Ts_Veh
  Divide1 : Product  Inputs=/*  SampleTime=UT.Ts_Veh
  Gain{8..11} (4 alike) : Gain
  Math Function : Math  Operator=square  SignedPower=on  SampleTime=UT.Ts_Veh
  Math Function1 : Math  Operator=square  SignedPower=on  SampleTime=UT.Ts_Veh
  Product : Product  SampleTime=UT.Ts_Veh
  Product1 : Product  SampleTime=UT.Ts_Veh
  Saturation : Saturate  UpperLimit=1  LowerLimit=-1
  Saturation{1,3..5} (4 alike) : Saturate  UpperLimit=15*3.14/180  LowerLimit=-15*3.14/180
  Saturation2 : Saturate  UpperLimit=1  LowerLimit=-1
  Sqrt : Sqrt  SampleTime=UT.Ts_Veh
  Switch : Switch  Criteria=u2 > Threshold  SaturateOnIntegerOverflow=off  InputSameDT=off
  Switch{1..4} (4 alike) : Switch  Threshold=2  SaturateOnIntegerOverflow=off  InputSameDT=off
  Vx{1..4} (4 alike) : InportShadow  Port=3
  Yaw Rate1 : InportShadow  Port=2
  alpha_fl: rad : Outport  VectorParamsAs1DForOutWhenUnconnected=off
  alpha_fr: rad : Outport  Port=2  VectorParamsAs1DForOutWhenUnconnected=off
  alpha_rl: rad : Outport  Port=3  VectorParamsAs1DForOutWhenUnconnected=off
  alpha_rr: rad : Outport  Port=4  VectorParamsAs1DForOutWhenUnconnected=off
  wires:
  Yaw Rate1/1 -> Product1/1
  Product1/1 -> Divide1/2
  Switch/1 -> Divide1/1, Divide/2
  Constant2/1 -> Switch/3
  Sqrt/1 -> Switch/1, Switch/2
  Add2/1 -> Switch2/1, Switch4/1
  Divide1/1 -> Add2/2
  Saturation2/1 -> Switch1/1
  Beta/1 -> Add1/1, Add4/1, Add2/1
  deltaFR1/1 -> Add4/3
  Divide/1 -> Add4/2, Add1/2
  Saturation/1 -> Switch3/1
  Vy/1 -> Math Function/1
  Add/1 -> Sqrt/1
  Math Function1/1 -> Add/2
  Math Function/1 -> Add/1
  deltaFL/1 -> Add1/3
  Gain11/1 -> alpha_rr: rad/1
  Gain10/1 -> alpha_rl: rad/1
  Gain8/1 -> alpha_fr: rad/1
  Gain9/1 -> alpha_fl: rad/1
  Saturation4/1 -> Gain11/1
  Saturation3/1 -> Gain10/1
  Saturation5/1 -> Gain8/1
  Saturation1/1 -> Gain9/1
  Switch4/1 -> Saturation4/1
  Vx4/1 -> Switch4/2
  Constant6/1 -> Switch4/3
  Switch2/1 -> Saturation3/1
  Vx3/1 -> Switch2/2
  Constant5/1 -> Switch2/3
  Switch1/1 -> Saturation5/1
  Vx2/1 -> Switch1/2
  Constant3/1 -> Switch1/3
  Switch3/1 -> Saturation1/1
  Vx1/1 -> Switch3/2
  Constant4/1 -> Switch3/3
  Add4/1 -> Saturation2/1
  Vx/1 -> Math Function1/1
  Add1/1 -> Saturation/1
  Constant1/1 -> Product1/2
  Product/1 -> Divide/1
  Yaw Rate/1 -> Product/1
  Constant/1 -> Product/2

== system EgoCarModel/PSG_first/Body Fixed Vehicle Dynamics/lamda slip ratio ==
  note: used to be divided by the max of abs of wheel vel or vwcosdelta
  omegafl : Inport
  omegafr : Inport  Port=2
  omegarl : Inport  Port=3
  omegarr : Inport  Port=4
  Vwfl : Inport  Port=5
  Vwfr : Inport  Port=6
  Vwrl : Inport  Port=7
  Vwrr : Inport  Port=8
  deltaFL : Inport  Port=9
  deltaFR : Inport  Port=10
  Abs{,1..7} (8 alike) : Abs  SaturateOnIntegerOverflow=off
  Constant : Constant  Value=UT.Rw
  Divide : Product  Inputs=*/  SampleTime=UT.Ts_Veh
  Divide1 : Product  Inputs=*/
  Divide2 : Product  Inputs=*/
  Divide3 : Product  Inputs=*/  SampleTime=UT.Ts_Veh
  Gain{,1..3} (4 alike) : Gain  Gain=0.1
  MinMax{,1..3} (4 alike) : MinMax  Function=max  Inputs=3
  Product{,1..5} (6 alike) : Product  SampleTime=UT.Ts_Veh
  Subtract : Sum  Inputs=+-  SampleTime=UT.Ts_Veh
  Subtract1 : Sum  Inputs=+-
  Subtract2 : Sum  Inputs=+-  SampleTime=UT.Ts_Veh
  Subtract3 : Sum  Inputs=+-  SampleTime=UT.Ts_Veh
  Trigonometric Function : Trigonometry  Operator=cos  SampleTime=UT.Ts_Veh
  Trigonometric Function1 : Trigonometry  Operator=cos
  VSlipMin : Constant  Value=UT.VSlipMin
  lamdafl : Outport  VectorParamsAs1DForOutWhenUnconnected=off
  lamdafr : Outport  Port=2  VectorParamsAs1DForOutWhenUnconnected=off
  lamdarl : Outport  Port=3  VectorParamsAs1DForOutWhenUnconnected=off
  lamdarr : Outport  Port=4  VectorParamsAs1DForOutWhenUnconnected=off
  wires:
  Gain3/1 -> lamdarr/1
  Gain1/1 -> lamdafr/1
  Product4/1 -> Abs1/1, Subtract/2
  deltaFR/1 -> Trigonometric Function1/1
  deltaFL/1 -> Trigonometric Function/1
  Vwrr/1 -> Subtract3/2, Abs7/1
  Gain2/1 -> lamdarl/1
  Gain/1 -> lamdafl/1
  Divide1/1 -> Gain1/1  "lamda_FR"
  Divide3/1 -> Gain3/1  "lamda_RR"
  Divide2/1 -> Gain2/1  "lamda_RL"
  MinMax3/1 -> Divide3/2
  Abs7/1 -> MinMax3/2
  Abs6/1 -> MinMax3/1
  MinMax2/1 -> Divide2/2
  Abs5/1 -> MinMax2/2
  Abs4/1 -> MinMax2/1
  MinMax1/1 -> Divide1/2
  Abs3/1 -> MinMax1/2
  Abs2/1 -> MinMax1/1
  MinMax/1 -> Divide/2
  Abs1/1 -> MinMax/2
  Abs/1 -> MinMax/1
  Subtract3/1 -> Divide3/1
  Subtract2/1 -> Divide2/1
  Subtract1/1 -> Divide1/1
  Subtract/1 -> Divide/1
  Vwrl/1 -> Subtract2/2, Abs5/1
  Vwfl/1 -> Product4/1
  Product5/1 -> Abs3/1, Subtract1/2
  Vwfr/1 -> Product5/1
  Trigonometric Function1/1 -> Product5/2
  Divide/1 -> Gain/1  "lamda_FL"
  Trigonometric Function/1 -> Product4/2
  Product3/1 -> Subtract3/1, Abs6/1
  Product2/1 -> Subtract2/1, Abs4/1
  Product1/1 -> Subtract1/1, Abs2/1
  Product/1 -> Subtract/1, Abs/1
  Constant/1 -> Product2/2, Product3/2, Product/2, Product1/2
  omegarr/1 -> Product3/1
  omegarl/1 -> Product2/1
  omegafr/1 -> Product1/1
  omegafl/1 -> Product/1
  VSlipMin/1 -> MinMax3/3, MinMax2/3, MinMax1/3, MinMax/3

== system EgoCarModel/PSG_first/Body Fixed Vehicle Dynamics/8dof_vehicle/4tyre_torque ==
  note: -20/Rw
  Tdf : Inport
  Tbfl : Inport  Port=2
  Tbfr : Inport  Port=3
  Tbrl : Inport  Port=4
  Tbrr : Inport  Port=5
  Fxfl : Inport  Port=6
  Fxfr : Inport  Port=7
  Fxrl : Inport  Port=8
  Fxrr : Inport  Port=9
  V_ini : Inport  Port=10
  Add2 : Sum  Inputs=--+
  Add3 : Sum  Inputs=+--
  Add4 : Sum  Inputs=--
  Add5 : Sum  Inputs=--
  Constant{,1..4} (5 alike) : Constant  Value=UT.Rw
  Discrete-Time Integrator{,1..3} (4 alike) : DiscreteIntegrator  InitialConditionSource=external  InitialCondition=UT.Veh_PSG_o(7)  SampleTime=UT.Ts_Veh  ICPrevOutput=DiscIntNeverNeededParam  ICPrevScaledInput=DiscIntNeverNeededParam
  Divide{,1..3} (4 alike) : Product  Inputs=*/
  Gain{1..3,5} (4 alike) : Gain  Gain=1/UT.Jw
  Product{,1..3} (4 alike) : Product
  Saturation{,1..3} (4 alike) : Saturate  UpperLimit=100/UT.Rw  LowerLimit=-20/UT.Rw
  omega_fl : Outport  VectorParamsAs1DForOutWhenUnconnected=off
  omega_fr : Outport  Port=2  VectorParamsAs1DForOutWhenUnconnected=off
  omega_rl : Outport  Port=3  VectorParamsAs1DForOutWhenUnconnected=off
  omega_rr : Outport  Port=4  VectorParamsAs1DForOutWhenUnconnected=off
  wires:
  Gain3/1 -> Discrete-Time Integrator3/1
  Product/1 -> Add2/1
  Tdf/1 -> Add3/1, Add2/3
  Constant/1 -> Product/2, Product3/1, Product2/1, Product1/1
  Product3/1 -> Add5/2
  Product2/1 -> Add4/2
  Tbfl/1 -> Add2/2
  Discrete-Time Integrator/1 -> Saturation/1
  Gain1/1 -> Discrete-Time Integrator1/1
  Discrete-Time Integrator1/1 -> Saturation1/1
  Gain2/1 -> Discrete-Time Integrator2/1
  Discrete-Time Integrator2/1 -> Saturation2/1
  Discrete-Time Integrator3/1 -> Saturation3/1
  Tbrl/1 -> Add4/1
  Add3/1 -> Gain1/1
  Add2/1 -> Gain5/1
  Add4/1 -> Gain2/1
  Add5/1 -> Gain3/1
  Gain5/1 -> Discrete-Time Integrator/1
  Fxfl/1 -> Product/1
  Fxfr/1 -> Product1/2
  Fxrl/1 -> Product2/2
  Fxrr/1 -> Product3/2
  Saturation/1 -> omega_fl/1
  Saturation1/1 -> omega_fr/1
  Saturation2/1 -> omega_rl/1
  Saturation3/1 -> omega_rr/1
  Product1/1 -> Add3/3
  Tbfr/1 -> Add3/2
  Tbrr/1 -> Add5/1
  Divide/1 -> Discrete-Time Integrator/2
  Constant1/1 -> Divide/2
  Constant2/1 -> Divide1/2
  Divide1/1 -> Discrete-Time Integrator1/2
  Divide2/1 -> Discrete-Time Integrator2/2
  Constant3/1 -> Divide2/2
  Constant4/1 -> Divide3/2
  Divide3/1 -> Discrete-Time Integrator3/2
  V_ini/1 -> Divide3/1, Divide2/1, Divide1/1, Divide/1
